simulink subsystem "forceToPWM"  (R2025b)
settings: Solver=VariableStepAuto  StartTime=0.0  StopTime=10.0  RelTol=1e-3
undefined symbols (not defined in the file or in its folder): force_table, pwm_list, voltage_list
settings Model: Creator=koryh  LastModifiedBy=koryh

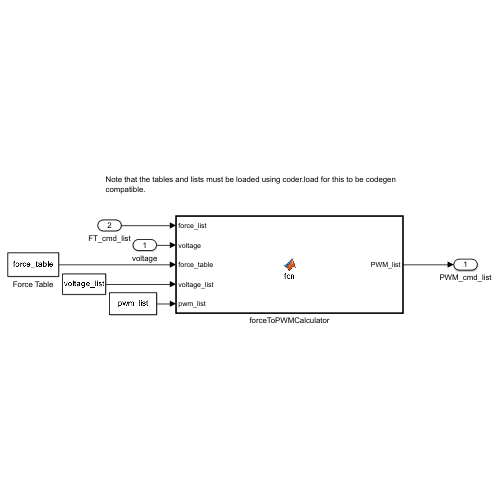
[thumbnail: Simulink's stored preview of the top-level diagram]
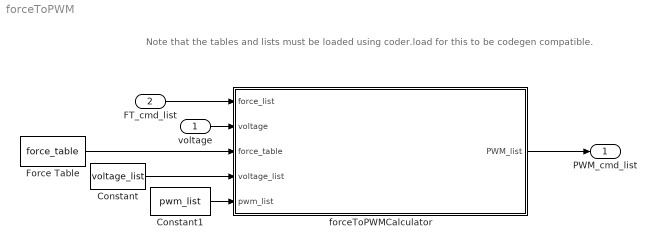
== system forceToPWM ==
  note: Note that the tables and lists must be loaded using coder.load for this to be codegen compatible.
  voltage : Inport
  FT_cmd_list : Inport  Port=2
  Constant : Constant  Value=voltage_list
  Constant1 : Constant  Value=pwm_list
  Force Table : Constant  Value=force_table
  forceToPWMCalculator : MATLAB Function  TreatAsAtomicUnit=on
  PWM_cmd_list : Outport
  wires:
  voltage/1 -> forceToPWMCalculator/2(voltage)
  Force Table/1 -> forceToPWMCalculator/3(force_table)
  forceToPWMCalculator/1(PWM_list) -> PWM_cmd_list/1
  Constant/1 -> forceToPWMCalculator/4(voltage_list)
  FT_cmd_list/1 -> forceToPWMCalculator/1(force_list)
  Constant1/1 -> forceToPWMCalculator/5(pwm_list)

== matlab function forceToPWM/forceToPWMCalculator ==
  data: force_list input; voltage input; PWM_list output; force_table input; voltage_list input; pwm_list input
function PWM_list = fcn(force_list,voltage,force_table,voltage_list,pwm_list)

PWM_list = forceToPWMCalculator(force_list,voltage,force_table,voltage_list,pwm_list);
